simulink library "WBIToolbox"  (Simulink 8.1)
settings: Solver=ode45  StartTime=0.0  StopTime=10.0  RelTol=1e-3
undefined symbols (not defined in the file or in its folder): localName, robotName
undefined symbols (not defined in the file): Ts, Tt
libraries: dspmtrx3 x5, WBCLibrary x5, simulink x1, dspsigops x1
(part 2 of 2)

== system WBIToolbox/wholeBodyModel/Dynamics/massMatrix/massMatrix ==
  q : Inport
  Constant : Constant  Value=0  OutDataTypeStr=int8  SampleTime=-1
  Constant1 : Constant  Value=zeros(25,1)  OutDataTypeStr=double  SampleTime=-1
  Constant3 : Constant  Value=zeros(31,1)  OutDataTypeStr=double  SampleTime=-1
  Constant4 : Constant  Value=zeros(31,1)  OutDataTypeStr=double  SampleTime=-1
  S-Function : S-Function  FunctionName=robotState  Parameters=val,robotname,localname  EnableBusSupport=off
  Terminator{,1..8} (9 alike) : Terminator
  massMatrix : Outport
  wires:
  S-Function/7 -> Terminator5/1
  S-Function/6 -> Terminator4/1
  S-Function/4 -> Terminator3/1
  S-Function/3 -> Terminator2/1
  S-Function/2 -> Terminator1/1
  S-Function/1 -> Terminator/1
  S-Function/5 -> massMatrix/1
  Constant1/1 -> S-Function/2
  Constant/1 -> S-Function/1
  S-Function/8 -> Terminator6/1
  S-Function/9 -> Terminator7/1
  S-Function/10 -> Terminator8/1
  q/1 -> S-Function/3
  Constant3/1 -> S-Function/4
  Constant4/1 -> S-Function/5

== system WBIToolbox/wholeBodyModel/Jacobians/Center of Mass Jacobian/Right Foot  Jacobian1 ==
  "Input Param. for forwardKinematics and  computeJacobians " : Constant  Value=2  OutDataTypeStr=int8  SampleTime=-1
  Input Param. for forwardKinematics and  computeJacobians 1 : Constant  Value=zeros(25,1)  OutDataTypeStr=double  SampleTime=-1
  Input Param. for forwardKinematics and  computeJacobians 2 : Constant  Value=zeros(25+16,1)  OutDataTypeStr=double  SampleTime=-1
  Input Param. for forwardKinematics and  computeJacobians 3 : Constant  Value=zeros(31,1)  OutDataTypeStr=double  SampleTime=-1
  Input Param. for forwardKinematics and  computeJacobians 4 : Constant  Value=zeros(31,1)  OutDataTypeStr=double  SampleTime=-1
  S-Function : S-Function  FunctionName=robotState  Parameters=val,robotname,localname  EnableBusSupport=off  mask{val=3, robotname=robotName, localname=localName}
      mask prompts: val "Value"; robotname "Robot Name (icub - icubSim)"; localname "Module Name"
  Terminator{1..2,4..5} (4 alike) : Terminator
  dqRad : Terminator
  massMatrix : Terminator
  massMatrix1 : Terminator
  qRad : Terminator
  x : Terminator
  Jacobian : Outport
  wires:
  S-Function/7 -> Terminator5/1
  S-Function/6 -> Terminator4/1
  S-Function/5 -> massMatrix/1
  S-Function/2 -> dqRad/1
  S-Function/1 -> qRad/1
  S-Function/3 -> x/1
  "Input Param. for forwardKinematics and  computeJacobians "/1 -> S-Function/1
  S-Function/4 -> Jacobian/1
  Input Param. for forwardKinematics and  computeJacobians 1/1 -> S-Function/2
  S-Function/8 -> massMatrix1/1
  S-Function/9 -> Terminator1/1
  S-Function/10 -> Terminator2/1
  Input Param. for forwardKinematics and  computeJacobians 2/1 -> S-Function/3
  Input Param. for forwardKinematics and  computeJacobians 3/1 -> S-Function/4
  Input Param. for forwardKinematics and  computeJacobians 4/1 -> S-Function/5

== system WBIToolbox/wholeBodyModel/Jacobians/Left Foot Jacobian/Left Foot  Jacobian1 ==
  "Input Param. for forwardKinematics and  computeJacobians " : Constant  OutDataTypeStr=int8
  Input Param. for forwardKinematics and  computeJacobians 1 : Constant  Value=zeros(25,1)  OutDataTypeStr=double  SampleTime=-1
  Input Param. for forwardKinematics and  computeJacobians 2 : Constant  Value=zeros(25+16,1)  OutDataTypeStr=double  SampleTime=-1
  Input Param. for forwardKinematics and  computeJacobians 3 : Constant  Value=zeros(31,1)  OutDataTypeStr=double  SampleTime=-1
  Input Param. for forwardKinematics and  computeJacobians 4 : Constant  Value=zeros(31,1)  OutDataTypeStr=double  SampleTime=-1
  S-Function : S-Function  FunctionName=robotState  Parameters=val,robotname,localname  EnableBusSupport=off  mask{val=3, robotname=robotName, localname=localName}
      mask prompts: val "Value"; robotname "Robot Name (icub - icubSim)"; localname "Module Name"
  Terminator1 : Terminator
  Terminator2 : Terminator
  Terminator3 : Terminator
  dqrad : Terminator
  dqrad1 : Terminator
  dqrad2 : Terminator
  massMatrix : Terminator
  massMatrix1 : Terminator
  qrad : Terminator
  Jacobian : Outport
  wires:
  Input Param. for forwardKinematics and  computeJacobians 1/1 -> S-Function/2
  S-Function/2 -> dqrad/1
  S-Function/1 -> qrad/1
  S-Function/3 -> Terminator1/1
  "Input Param. for forwardKinematics and  computeJacobians "/1 -> S-Function/1
  S-Function/4 -> Jacobian/1
  S-Function/5 -> massMatrix/1
  S-Function/6 -> Terminator3/1
  S-Function/7 -> dqrad1/1
  S-Function/8 -> massMatrix1/1
  S-Function/9 -> Terminator2/1
  S-Function/10 -> dqrad2/1
  Input Param. for forwardKinematics and  computeJacobians 2/1 -> S-Function/3
  Input Param. for forwardKinematics and  computeJacobians 3/1 -> S-Function/4
  Input Param. for forwardKinematics and  computeJacobians 4/1 -> S-Function/5

== system WBIToolbox/wholeBodyModel/Jacobians/Left Hand Jacobian/Left Hand  Jacobian ==
  "Input Param. for forwardKinematics and  computeJacobians " : Constant  Value=4  OutDataTypeStr=int8
  Input Param. for forwardKinematics and  computeJacobians 1 : Constant  Value=zeros(25,1)  OutDataTypeStr=double  SampleTime=-1
  Input Param. for forwardKinematics and  computeJacobians 2 : Constant  Value=zeros(25+16,1)  OutDataTypeStr=double  SampleTime=-1
  Input Param. for forwardKinematics and  computeJacobians 3 : Constant  Value=zeros(31,1)  OutDataTypeStr=double  SampleTime=-1
  Input Param. for forwardKinematics and  computeJacobians 4 : Constant  Value=zeros(31,1)  OutDataTypeStr=double  SampleTime=-1
  S-Function : S-Function  FunctionName=robotState  Parameters=val,robotname,localname  EnableBusSupport=off  mask{val=3, robotname=robotName, localname=localName}
      mask prompts: val "Value"; robotname "Robot Name (icub - icubSim)"; localname "Module Name"
  Terminator1 : Terminator
  Terminator2 : Terminator
  Terminator3 : Terminator
  dqrad : Terminator
  dqrad1 : Terminator
  dqrad2 : Terminator
  massMatrix : Terminator
  massMatrix1 : Terminator
  qrad : Terminator
  Jacobian : Outport
  wires:
  Input Param. for forwardKinematics and  computeJacobians 4/1 -> S-Function/5
  Input Param. for forwardKinematics and  computeJacobians 3/1 -> S-Function/4
  Input Param. for forwardKinematics and  computeJacobians 2/1 -> S-Function/3
  S-Function/10 -> dqrad2/1
  S-Function/9 -> Terminator2/1
  S-Function/8 -> massMatrix1/1
  S-Function/7 -> dqrad1/1
  S-Function/6 -> Terminator3/1
  S-Function/5 -> massMatrix/1
  S-Function/4 -> Jacobian/1
  "Input Param. for forwardKinematics and  computeJacobians "/1 -> S-Function/1
  S-Function/3 -> Terminator1/1
  S-Function/1 -> qrad/1
  S-Function/2 -> dqrad/1
  Input Param. for forwardKinematics and  computeJacobians 1/1 -> S-Function/2

== system WBIToolbox/wholeBodyModel/Jacobians/Right Foot Jacobian/Right Foot  Jacobian1 ==
  "Input Param. for forwardKinematics and  computeJacobians " : Constant  Value=0  OutDataTypeStr=int8  SampleTime=-1
  Input Param. for forwardKinematics and  computeJacobians 1 : Constant  Value=zeros(25,1)  OutDataTypeStr=double  SampleTime=-1
  Input Param. for forwardKinematics and  computeJacobians 2 : Constant  Value=zeros(25+16,1)  OutDataTypeStr=double  SampleTime=-1
  Input Param. for forwardKinematics and  computeJacobians 3 : Constant  Value=zeros(31,1)  OutDataTypeStr=double  SampleTime=-1
  Input Param. for forwardKinematics and  computeJacobians 4 : Constant  Value=zeros(31,1)  OutDataTypeStr=double  SampleTime=-1
  S-Function : S-Function  FunctionName=robotState  Parameters=val,robotname,localname  EnableBusSupport=off  mask{val=3, robotname=robotName, localname=localName}
      mask prompts: val "Value"; robotname "Robot Name (icub - icubSim)"; localname "Module Name"
  Terminator{1..5} (5 alike) : Terminator
  dqRad : Terminator
  massMatrix : Terminator
  qRad : Terminator
  x : Terminator
  Jacobian : Outport
  wires:
  Input Param. for forwardKinematics and  computeJacobians 1/1 -> S-Function/2
  S-Function/4 -> Jacobian/1
  "Input Param. for forwardKinematics and  computeJacobians "/1 -> S-Function/1
  S-Function/3 -> x/1
  S-Function/1 -> qRad/1
  S-Function/2 -> dqRad/1
  S-Function/5 -> massMatrix/1
  S-Function/6 -> Terminator4/1
  S-Function/7 -> Terminator5/1
  S-Function/8 -> Terminator1/1
  S-Function/9 -> Terminator2/1
  S-Function/10 -> Terminator3/1
  Input Param. for forwardKinematics and  computeJacobians 2/1 -> S-Function/3
  Input Param. for forwardKinematics and  computeJacobians 3/1 -> S-Function/4
  Input Param. for forwardKinematics and  computeJacobians 4/1 -> S-Function/5

== system WBIToolbox/wholeBodyModel/Jacobians/Right Hand Jacobian/Right Hand Jacobian ==
  "Input Param. for forwardKinematics and  computeJacobians " : Constant  Value=3  OutDataTypeStr=int8  SampleTime=-1
  Input Param. for forwardKinematics and  computeJacobians 1 : Constant  Value=zeros(25,1)  OutDataTypeStr=double  SampleTime=-1
  Input Param. for forwardKinematics and  computeJacobians 2 : Constant  Value=zeros(25+16,1)  OutDataTypeStr=double  SampleTime=-1
  Input Param. for forwardKinematics and  computeJacobians 3 : Constant  Value=zeros(31,1)  OutDataTypeStr=double  SampleTime=-1
  Input Param. for forwardKinematics and  computeJacobians 4 : Constant  Value=zeros(31,1)  OutDataTypeStr=double  SampleTime=-1
  S-Function : S-Function  FunctionName=robotState  Parameters=val,robotname,localname  EnableBusSupport=off  mask{val=3, robotname=robotName, localname=localName}
      mask prompts: val "Value"; robotname "Robot Name (icub - icubSim)"; localname "Module Name"
  Terminator{1..5} (5 alike) : Terminator
  dqRad : Terminator
  massMatrix : Terminator
  qRad : Terminator
  x : Terminator
  Jacobian : Outport
  wires:
  Input Param. for forwardKinematics and  computeJacobians 4/1 -> S-Function/5
  Input Param. for forwardKinematics and  computeJacobians 3/1 -> S-Function/4
  Input Param. for forwardKinematics and  computeJacobians 2/1 -> S-Function/3
  S-Function/10 -> Terminator3/1
  S-Function/9 -> Terminator2/1
  S-Function/8 -> Terminator1/1
  S-Function/7 -> Terminator5/1
  S-Function/6 -> Terminator4/1
  S-Function/5 -> massMatrix/1
  S-Function/2 -> dqRad/1
  S-Function/1 -> qRad/1
  S-Function/3 -> x/1
  "Input Param. for forwardKinematics and  computeJacobians "/1 -> S-Function/1
  S-Function/4 -> Jacobian/1
  Input Param. for forwardKinematics and  computeJacobians 1/1 -> S-Function/2

== matlab function Utilities/baseVelocity/MATLAB Function ==
  data: JcIn input double; y output double; qD input double
function y = fcn(JcIn, qD)
%#codegen
y = -pinv(JcIn(:,1:6))*JcIn(:,7:end)*qD;

== matlab function Utilities/DampPinv/Damped Pseudo Inverse ==
  data: mat input double; DPinv output double; sigma input double
function DPinv  = fcn(mat,sigma)
% Economody size svd of mat
[U,S,V] = svd(mat,'econ');
% Damped version of S with sigma
S(S>sigma)=S(S>sigma)./((S(S>sigma)).^2+sigma^2);
% Damped pseudoinverse
DPinv = V*pinv(S)*U';

== matlab function Utilities/TruncPinv/Truncated PseudoInverse ==
  data: mat input double; TPinv output double; tol input double
function TPinv  = fcn(mat,tol)
%#codegen
[U,S,V] = svd(mat,'econ');
% Setting to zero value
% Setting to 1/S(i,i) singular values greater than tol
 S(S>tol)=1./S(S>tol);
 TPinv = V*pinv(S)*U';
